simulink model "HARMALYZE_model_simulink"  (R2019b)
settings: Solver=VariableStepAuto  StartTime=0.0  StopTime=2.3  RelTol=1e-3
libraries: powerlib_meascontrol x1
(part 1 of 2)
settings Model: Creator=91850  LastModifiedBy=91850

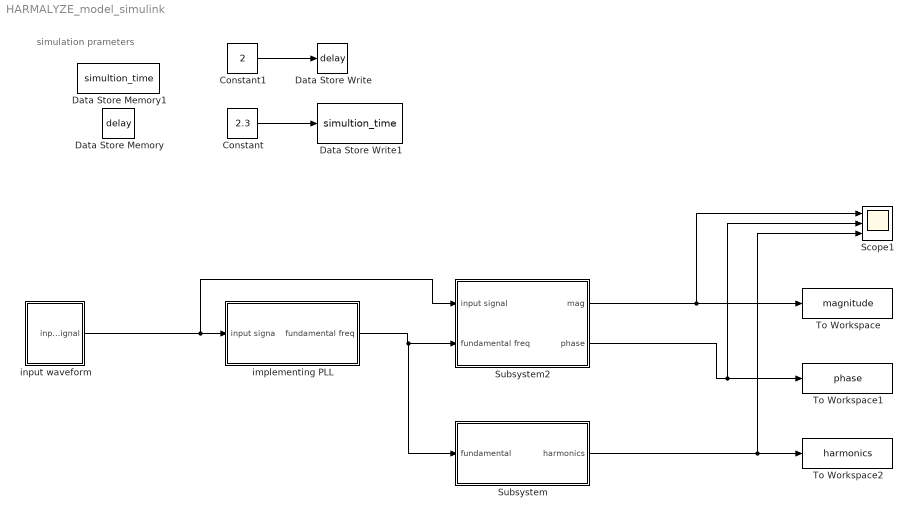
== system HARMALYZE_model_simulink ==
  note: simulation prameters
  Constant : Constant  Value=2.3
  Constant1 : Constant  Value=2
  Data Store Write : DataStoreWrite  DataStoreName=delay
  Data Store Write1 : DataStoreWrite  DataStoreName=simultion_time
  Data Store Memory : DataStoreMemory  DataStoreName=delay  ReadBeforeWriteMsg=warning  WriteAfterWriteMsg=warning  WriteAfterReadMsg=warning  ShowAdditionalParam=off
  Data Store Memory1 : DataStoreMemory  DataStoreName=simultion_time  ReadBeforeWriteMsg=warning  WriteAfterWriteMsg=warning  WriteAfterReadMsg=warning  ShowAdditionalParam=off
  Scope1 : Scope  NumInputPorts=3
  Subsystem : Subsystem
  Subsystem2 : Subsystem
  To Workspace : ToWorkspace  VariableName=magnitude  SaveFormat=Timeseries  SampleTime=-1
  To Workspace1 : ToWorkspace  VariableName=phase  SaveFormat=Timeseries  SampleTime=-1
  To Workspace2 : ToWorkspace  VariableName=harmonics  SaveFormat=Timeseries  SampleTime=-1
  implementing PLL : Subsystem
  input waveform : Subsystem
  wires:
  Constant1/1 -> Data Store Write/1
  Constant/1 -> Data Store Write1/1
  Subsystem2/1("mag ") -> Scope1/1, To Workspace/1
  Subsystem2/2(phase) -> Scope1/2, To Workspace1/1
  input waveform/1(input signal) -> Subsystem2/1(input signal), implementing PLL/1(input signa)
  implementing PLL/1(fundamental freq) -> Subsystem/1(fundamental), Subsystem2/2(fundamental freq)
  Subsystem/1(harmonics) -> Scope1/3, To Workspace2/1

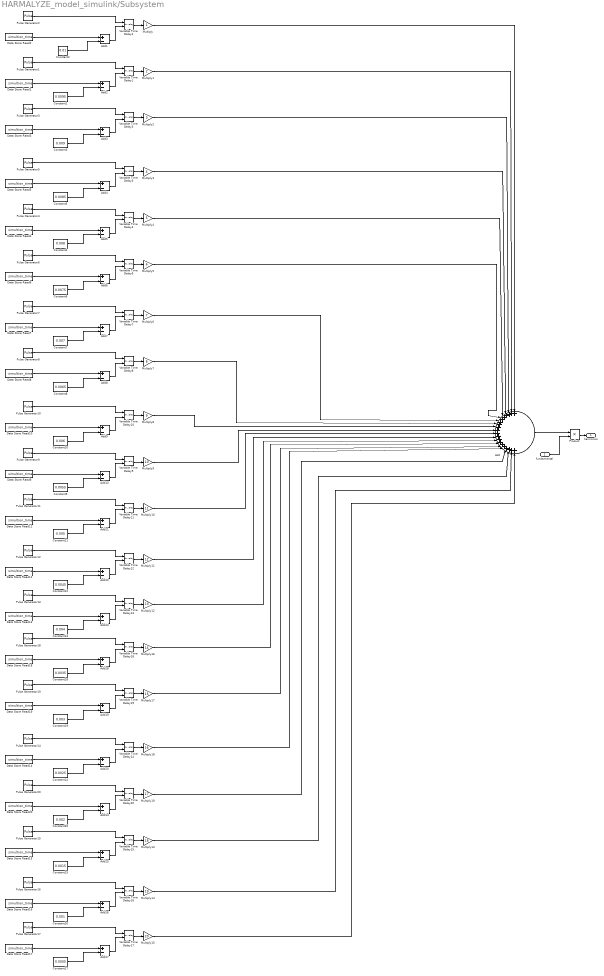
== system HARMALYZE_model_simulink/Subsystem ==
  fundamental : Inport
  Add : Sum  Inputs=20
  Add{1..20} (20 alike) : Sum  Inputs=+-
  Constant1 : Constant  Value=0.0095
  Constant10 : Constant  Value=0.006
  Constant11 : Constant  Value=0.005
  Constant12 : Constant  Value=0.0045
  Constant13 : Constant  Value=0.004
  Constant14 : Constant  Value=0.0025
  Constant15 : Constant  Value=0.0015
  Constant16 : Constant  Value=0.001
  Constant17 : Constant  Value=0.0005
  Constant18 : Constant  Value=0.0035
  Constant19 : Constant  Value=0.003
  Constant2 : Constant  Value=0.01
  Constant20 : Constant  Value=0.002
  Constant3 : Constant  Value=0.009
  Constant4 : Constant  Value=0.008
  Constant5 : Constant  Value=0.0085
  Constant6 : Constant  Value=0.0075
  Constant7 : Constant  Value=0.007
  Constant8 : Constant  Value=0.0065
  Constant9 : Constant  Value=0.0055
  Data Store Read{1..20} (20 alike) : DataStoreRead  DataStoreName=simultion_time
  Multiply : Gain
  Multiply1 : Gain  Gain=2
  Multiply10 : Gain  Gain=11
  Multiply11 : Gain  Gain=12
  Multiply12 : Gain  Gain=13
  Multiply13 : Gain  Gain=18
  Multiply14 : Gain  Gain=19
  Multiply15 : Gain  Gain=20
  Multiply16 : Gain  Gain=14
  Multiply17 : Gain  Gain=15
  Multiply18 : Gain  Gain=16
  Multiply19 : Gain  Gain=17
  Multiply2 : Gain  Gain=3
  Multiply3 : Gain  Gain=4
  Multiply4 : Gain  Gain=5
  Multiply5 : Gain  Gain=6
  Multiply6 : Gain  Gain=7
  Multiply7 : Gain  Gain=8
  Multiply8 : Gain  Gain=9
  Multiply9 : Gain  Gain=10
  Product : Product
  Pulse Generator{1..20} (20 alike) : DiscretePulseGenerator  PulseType=Time based  Period=1  PulseWidth=0.01
  Variable Time Delay{1..20} (20 alike) : VariableTransportDelay  MaximumDelay=10
  harmonics : Outport
  wires:
  Add1/1 -> Variable Time Delay2/2
  Data Store Read2/1 -> Add1/1
  Pulse Generator2/1 -> Variable Time Delay2/1
  Product/1 -> harmonics/1
  Constant2/1 -> Add1/2
  Constant1/1 -> Add2/2
  Pulse Generator1/1 -> Variable Time Delay1/1
  Data Store Read1/1 -> Add2/1
  Add2/1 -> Variable Time Delay1/2
  Add/1 -> Product/1
  fundamental/1 -> Product/2
  Variable Time Delay2/1 -> Multiply/1
  Variable Time Delay1/1 -> Multiply1/1
  Variable Time Delay3/1 -> Multiply2/1
  Add3/1 -> Variable Time Delay3/2
  Data Store Read3/1 -> Add3/1
  Pulse Generator3/1 -> Variable Time Delay3/1
  Constant3/1 -> Add3/2
  Constant6/1 -> Add6/2
  Pulse Generator6/1 -> Variable Time Delay6/1
  Data Store Read6/1 -> Add6/1
  Add6/1 -> Variable Time Delay6/2
  Variable Time Delay6/1 -> Multiply5/1
  Variable Time Delay4/1 -> Multiply4/1
  Variable Time Delay5/1 -> Multiply3/1
  Add5/1 -> Variable Time Delay4/2
  Data Store Read4/1 -> Add5/1
  Pulse Generator4/1 -> Variable Time Delay4/1
  Constant4/1 -> Add5/2
  Constant5/1 -> Add4/2
  Pulse Generator5/1 -> Variable Time Delay5/1
  Data Store Read5/1 -> Add4/1
  Add4/1 -> Variable Time Delay5/2
  Add9/1 -> Variable Time Delay10/2
  Data Store Read10/1 -> Add9/1
  Pulse Generator10/1 -> Variable Time Delay10/1
  Constant10/1 -> Add9/2
  Constant9/1 -> Add10/2
  Pulse Generator9/1 -> Variable Time Delay9/1
  Data Store Read9/1 -> Add10/1
  Add10/1 -> Variable Time Delay9/2
  Variable Time Delay10/1 -> Multiply8/1
  Variable Time Delay9/1 -> Multiply9/1
  Variable Time Delay11/1 -> Multiply10/1
  Add11/1 -> Variable Time Delay11/2
  Data Store Read11/1 -> Add11/1
  Pulse Generator11/1 -> Variable Time Delay11/1
  Constant11/1 -> Add11/2
  Constant8/1 -> Add8/2
  Pulse Generator8/1 -> Variable Time Delay8/1
  Data Store Read8/1 -> Add8/1
  Add8/1 -> Variable Time Delay8/2
  Variable Time Delay8/1 -> Multiply7/1
  Variable Time Delay7/1 -> Multiply6/1
  Add7/1 -> Variable Time Delay7/2
  Data Store Read7/1 -> Add7/1
  Pulse Generator7/1 -> Variable Time Delay7/1
  Constant7/1 -> Add7/2
  Constant12/1 -> Add12/2
  Pulse Generator12/1 -> Variable Time Delay12/1
  Data Store Read12/1 -> Add12/1
  Add12/1 -> Variable Time Delay12/2
  Variable Time Delay12/1 -> Multiply11/1
  Variable Time Delay13/1 -> Multiply12/1
  Add13/1 -> Variable Time Delay13/2
  Data Store Read13/1 -> Add13/1
  Pulse Generator13/1 -> Variable Time Delay13/1
  Constant13/1 -> Add13/2
  Constant17/1 -> Add17/2
  Pulse Generator17/1 -> Variable Time Delay17/1
  Data Store Read17/1 -> Add17/1
  Add17/1 -> Variable Time Delay17/2
  Variable Time Delay17/1 -> Multiply15/1
  Variable Time Delay16/1 -> Multiply14/1
  Add16/1 -> Variable Time Delay16/2
  Data Store Read16/1 -> Add16/1
  Pulse Generator16/1 -> Variable Time Delay16/1
  Constant16/1 -> Add16/2
  Constant18/1 -> Add18/2
  Pulse Generator18/1 -> Variable Time Delay18/1
  Data Store Read18/1 -> Add18/1
  Add18/1 -> Variable Time Delay18/2
  Variable Time Delay18/1 -> Multiply16/1
  Variable Time Delay19/1 -> Multiply17/1
  Add19/1 -> Variable Time Delay19/2
  Data Store Read19/1 -> Add19/1
  Pulse Generator19/1 -> Variable Time Delay19/1
  Constant19/1 -> Add19/2
  Constant15/1 -> Add15/2
  Pulse Generator15/1 -> Variable Time Delay15/1
  Data Store Read15/1 -> Add15/1
  Add15/1 -> Variable Time Delay15/2
  Variable Time Delay15/1 -> Multiply13/1
  Variable Time Delay20/1 -> Multiply19/1
  Variable Time Delay14/1 -> Multiply18/1
  Add14/1 -> Variable Time Delay20/2
  Data Store Read20/1 -> Add14/1
  Pulse Generator20/1 -> Variable Time Delay20/1
  Constant20/1 -> Add14/2
  Constant14/1 -> Add20/2
  Pulse Generator14/1 -> Variable Time Delay14/1
  Data Store Read14/1 -> Add20/1
  Add20/1 -> Variable Time Delay14/2
  Multiply/1 -> Add/1
  Multiply1/1 -> Add/2
  Multiply2/1 -> Add/3
  Multiply3/1 -> Add/4
  Multiply4/1 -> Add/5
  Multiply5/1 -> Add/6
  Multiply6/1 -> Add/7
  Multiply7/1 -> Add/8
  Multiply8/1 -> Add/9
  Multiply9/1 -> Add/10
  Multiply10/1 -> Add/11
  Multiply11/1 -> Add/12
  Multiply12/1 -> Add/13
  Multiply16/1 -> Add/14
  Multiply17/1 -> Add/15
  Multiply18/1 -> Add/16
  Multiply19/1 -> Add/17
  Multiply13/1 -> Add/18
  Multiply14/1 -> Add/19
  Multiply15/1 -> Add/20

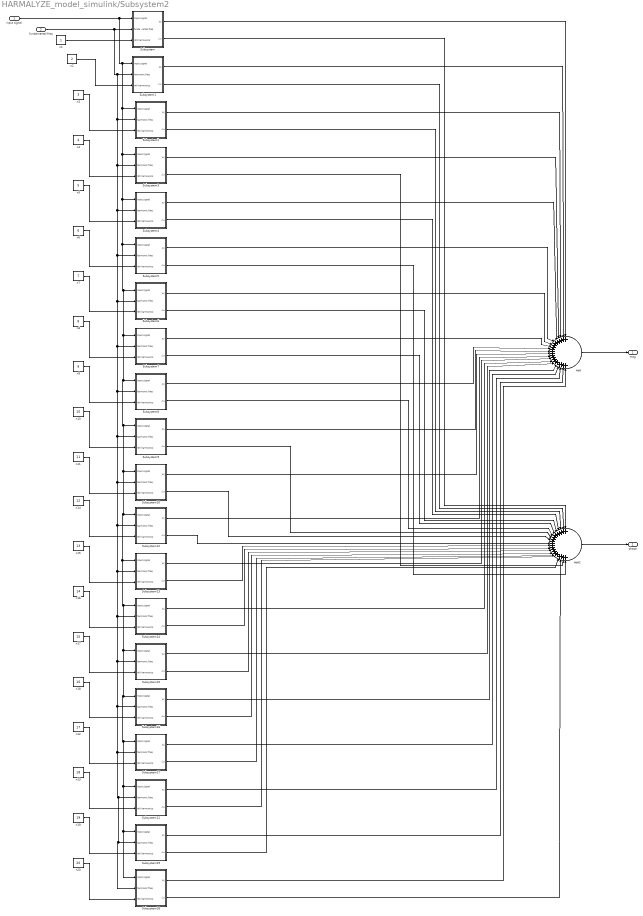
== system HARMALYZE_model_simulink/Subsystem2 ==
  input signal : Inport
  fundamental freq : Inport  Port=2
  Add : Sum  Inputs=20
  Add2 : Sum  Inputs=20
  Subsystem : Subsystem
  Subsystem1 : Subsystem
  Subsystem10 : Subsystem
  Subsystem11 : Subsystem
  Subsystem12 : Subsystem
  Subsystem13 : Subsystem
  Subsystem14 : Subsystem
  Subsystem15 : Subsystem
  Subsystem16 : Subsystem
  Subsystem17 : Subsystem
  Subsystem18 : Subsystem
  Subsystem19 : Subsystem
  Subsystem2 : Subsystem
  Subsystem3 : Subsystem
  Subsystem4 : Subsystem
  Subsystem5 : Subsystem
  Subsystem6 : Subsystem
  Subsystem7 : Subsystem
  Subsystem8 : Subsystem
  Subsystem9 : Subsystem
  n1 : Constant
  n10 : Constant  Value=10
  n11 : Constant  Value=11
  n12 : Constant  Value=17
  n13 : Constant  Value=18
  n14 : Constant  Value=12
  n15 : Constant  Value=13
  n16 : Constant  Value=14
  n17 : Constant  Value=15
  n18 : Constant  Value=16
  n19 : Constant  Value=19
  n2 : Constant  Value=2
  n20 : Constant  Value=20
  n3 : Constant  Value=3
  n4 : Constant  Value=4
  n5 : Constant  Value=5
  n6 : Constant  Value=6
  n7 : Constant  Value=7
  n8 : Constant  Value=8
  n9 : Constant  Value=9
  "mag " : Outport
  phase : Outport  Port=2
  wires:
  Subsystem/1(|u|) -> Add/1
  n1/1 -> Subsystem/3(nth harmonics)
  n2/1 -> Subsystem1/3(nth harmonics)
  Subsystem1/1(|u|) -> Add/2
  Subsystem2/1(|u|) -> Add/3
  n3/1 -> Subsystem2/3(nth harmonics)
  n4/1 -> Subsystem3/3(nth harmonics)
  Subsystem3/1(|u|) -> Add/4
  n5/1 -> Subsystem4/3(nth harmonics)
  Subsystem4/1(|u|) -> Add/5
  n6/1 -> Subsystem5/3(nth harmonics)
  Subsystem5/1(|u|) -> Add/6
  n7/1 -> Subsystem6/3(nth harmonics)
  Subsystem6/1(|u|) -> Add/7
  n8/1 -> Subsystem7/3(nth harmonics)
  Subsystem7/1(|u|) -> Add/8
  n11/1 -> Subsystem10/3(nth harmonics)
  Subsystem9/1(|u|) -> Add/10
  n10/1 -> Subsystem9/3(nth harmonics)
  Subsystem8/1(|u|) -> Add/9
  n9/1 -> Subsystem8/3(nth harmonics)
  n18/1 -> Subsystem16/3(nth harmonics)
  Subsystem16/1(|u|) -> Add/16
  n12/1 -> Subsystem17/3(nth harmonics)
  n13/1 -> Subsystem11/3(nth harmonics)
  Subsystem15/1(|u|) -> Add/15
  n17/1 -> Subsystem15/3(nth harmonics)
  Subsystem14/1(|u|) -> Add/14
  n16/1 -> Subsystem14/3(nth harmonics)
  Subsystem13/1(|u|) -> Add/13
  n15/1 -> Subsystem13/3(nth harmonics)
  Subsystem12/1(|u|) -> Add/12
  n14/1 -> Subsystem12/3(nth harmonics)
  fundamental freq/1 -> Subsystem9/2(harmonic freq), Subsystem13/2(harmonic freq), Subsystem14/2(harmonic freq), Subsystem15/2(harmonic freq), Subsystem16/2(harmonic freq), Subsystem18/2(harmonic freq), Subsystem19/2(harmonic freq), Subsystem11/2(harmonic freq), Subsystem17/2(harmonic freq), Subsystem12/2(harmonic freq), Subsystem10/2(harmonic freq), Subsystem8/2(harmonic freq), Subsystem7/2(harmonic freq), Subsystem6/2(harmonic freq), Subsystem5/2(harmonic freq), Subsystem4/2(harmonic freq), Subsystem3/2(harmonic freq), Subsystem2/2(harmonic freq), Subsystem1/2(harmonic freq), Subsystem/2(fundamental freq)
  n20/1 -> Subsystem18/3(nth harmonics)
  input signal/1 -> Subsystem9/1(input signal), Subsystem13/1(input signal), Subsystem14/1(input signal), Subsystem15/1(input signal), Subsystem16/1(input signal), Subsystem19/1(input signal), Subsystem18/1(input signal), Subsystem11/1(input signal), Subsystem17/1(input signal), Subsystem12/1(input signal), Subsystem10/1(input signal), Subsystem8/1(input signal), Subsystem7/1(input signal), Subsystem6/1(input signal), Subsystem5/1(input signal), Subsystem4/1(input signal), Subsystem3/1(input signal), Subsystem2/1(input signal), Subsystem1/1(input signal), Subsystem/1(input signal)
  n19/1 -> Subsystem19/3(nth harmonics)
  Subsystem10/1(|u|) -> Add/11
  Subsystem17/1(|u|) -> Add/17
  Subsystem11/1(|u|) -> Add/18
  Subsystem19/1(|u|) -> Add/19
  Subsystem18/1(|u|) -> Add/20
  Subsystem/2(∠u) -> Add2/1
  Subsystem1/2(∠u) -> Add2/2
  Subsystem2/2(∠u) -> Add2/3
  Subsystem4/2(∠u) -> Add2/4
  Subsystem6/2(∠u) -> Add2/5
  Subsystem9/2(∠u) -> Add2/8
  Subsystem12/2(∠u) -> Add2/10
  Subsystem10/2(∠u) -> Add2/9
  Subsystem7/2(∠u) -> Add2/6
  Subsystem8/2(∠u) -> Add2/7
  Subsystem13/2(∠u) -> Add2/11
  Subsystem14/2(∠u) -> Add2/12
  Subsystem15/2(∠u) -> Add2/13
  Subsystem16/2(∠u) -> Add2/14
  Subsystem17/2(∠u) -> Add2/15
  Subsystem11/2(∠u) -> Add2/16
  Subsystem19/2(∠u) -> Add2/17
  Subsystem18/2(∠u) -> Add2/18
  Subsystem3/2(∠u) -> Add2/19
  Subsystem5/2(∠u) -> Add2/20
  Add/1 -> "mag "/1
  Add2/1 -> phase/1

== system HARMALYZE_model_simulink/implementing PLL ==
  input signa : Inport
  Clock1 : Clock
  Data Store Read : DataStoreRead  DataStoreName=delay
  If Action Subsystem : Subsystem  TreatAsAtomicUnit=on
  If1 : If  NumInputs=2  IfExpression=u1 == u2  ShowElse=off
  pll : powerlib_meascontrol/PLL/PLL  Fmin=10  Par_Init=[0, 40]  ParK=[180, 3200, 1]  TcD=1e-4  MaxRateChangeFreq=10  FilterCutOffFreq=25  Ts=0  AGC=on
      settings: SourceProductName=Simscape Electrical  SourceProductBaseCode=PS
  fundamental freq : Outport
  wires:
  If Action Subsystem/1(Out1) -> fundamental freq/1
  If1/1 -> If Action Subsystem/Action
  Clock1/1 -> If1/1
  pll/1 -> If Action Subsystem/1(In1)
  Data Store Read/1 -> If1/2
  input signa/1 -> pll/1

== system HARMALYZE_model_simulink/input waveform ==
  Add1 : Sum  Inputs=5
  "fundamental " : SignalGenerator  Amplitude=10  Frequency=50
  harmonic 1 : SignalGenerator  Amplitude=5  Frequency=100
  harmonic 2 : SignalGenerator  Amplitude=3  Frequency=150
  harmonic 3 : SignalGenerator  Amplitude=2  Frequency=200
  harmonic 4 : SignalGenerator  Frequency=250
  input signal : Outport
  wires:
  harmonic 1/1 -> Add1/2
  harmonic 2/1 -> Add1/3
  Add1/1 -> input signal/1
  "fundamental "/1 -> Add1/1
  harmonic 3/1 -> Add1/4
  harmonic 4/1 -> Add1/5

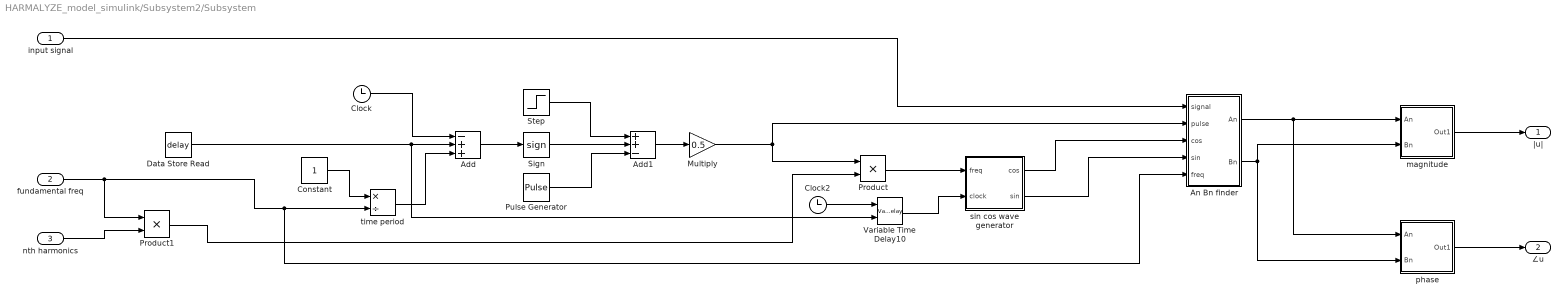
== system HARMALYZE_model_simulink/Subsystem2/Subsystem ==
  input signal : Inport
  fundamental freq : Inport  Port=2
  nth harmonics : Inport  Port=3
  Add : Sum  Inputs=-++
  Add1 : Sum  Inputs=++-
  An Bn finder : Subsystem
  Clock : Clock
  Clock2 : Clock
  Constant : Constant
  Data Store Read : DataStoreRead  DataStoreName=delay
  Multiply : Gain  Gain=0.5
  Product : Product
  Product1 : Product
  Pulse Generator : DiscretePulseGenerator  PulseType=Time based  Period=4  PulseWidth=50
  Sign : Signum
  Step : Step  Time=2  SampleTime=0
  Variable Time Delay10 : VariableTransportDelay  MaximumDelay=10
  magnitude : Subsystem
  phase : Subsystem
  sin cos wave generator : Subsystem
  "time period " : Product  Inputs=*/
  |u| : Outport
  ∠u : Outport  Port=2
  wires:
  input signal/1 -> An Bn finder/1(signal)
  sin cos wave generator/2(sin) -> An Bn finder/4(sin)
  sin cos wave generator/1(cos) -> An Bn finder/3(cos)
  Variable Time Delay10/1 -> sin cos wave generator/2(clock)
  "time period "/1 -> Add/3
  Data Store Read/1 -> Variable Time Delay10/2, Add/2
  Multiply/1 -> Product/1, An Bn finder/2(pulse)
  Product/1 -> sin cos wave generator/1(freq)
  Clock/1 -> Add/1
  Add/1 -> Sign/1
  Constant/1 -> "time period "/1
  Step/1 -> Add1/1
  Sign/1 -> Add1/2
  Pulse Generator/1 -> Add1/3
  Clock2/1 -> Variable Time Delay10/1
  Add1/1 -> Multiply/1
  Product1/1 -> Product/2
  An Bn finder/2(Bn) -> phase/2(Bn), magnitude/2(Bn)
  An Bn finder/1(An) -> phase/1(An), magnitude/1(An)
  magnitude/1(Out1) -> |u|/1
  phase/1(Out1) -> ∠u/1
  nth harmonics/1 -> Product1/2
  fundamental freq/1 -> Product1/1, An Bn finder/5("freq "), "time period "/2

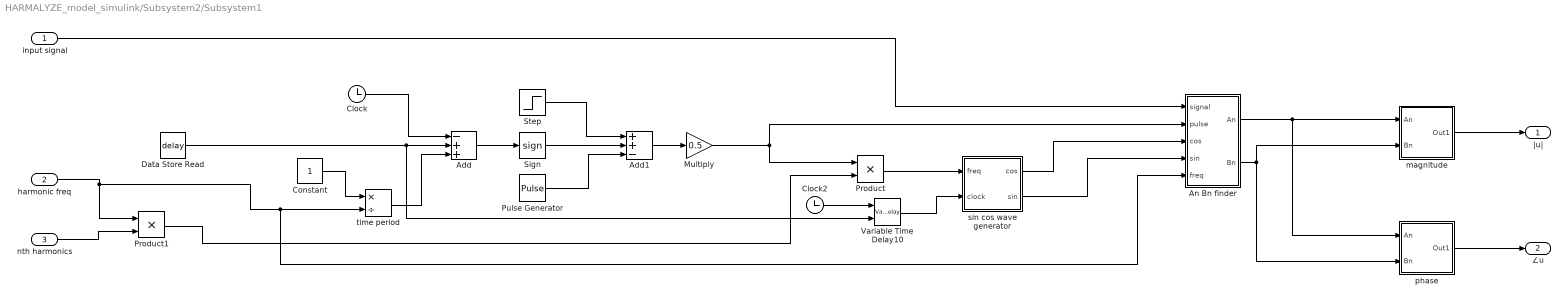
== system HARMALYZE_model_simulink/Subsystem2/Subsystem1 ==
  input signal : Inport
  harmonic freq : Inport  Port=2
  nth harmonics : Inport  Port=3
  Add : Sum  Inputs=-++
  Add1 : Sum  Inputs=++-
  An Bn finder : Subsystem
  Clock : Clock
  Clock2 : Clock
  Constant : Constant
  Data Store Read : DataStoreRead  DataStoreName=delay
  Multiply : Gain  Gain=0.5
  Product : Product
  Product1 : Product
  Pulse Generator : DiscretePulseGenerator  PulseType=Time based  Period=4  PulseWidth=50
  Sign : Signum
  Step : Step  Time=2  SampleTime=0
  Variable Time Delay10 : VariableTransportDelay  MaximumDelay=10
  magnitude : Subsystem
  phase : Subsystem
  sin cos wave generator : Subsystem
  "time period " : Product  Inputs=*/
  |u| : Outport
  ∠u : Outport  Port=2
  wires:
  harmonic freq/1 -> Product1/1, "time period "/2, An Bn finder/5("freq ")
  nth harmonics/1 -> Product1/2
  phase/1(Out1) -> ∠u/1
  magnitude/1(Out1) -> |u|/1
  An Bn finder/1(An) -> magnitude/1(An), phase/1(An)
  An Bn finder/2(Bn) -> magnitude/2(Bn), phase/2(Bn)
  Product1/1 -> Product/2
  Add1/1 -> Multiply/1
  Clock2/1 -> Variable Time Delay10/1
  Pulse Generator/1 -> Add1/3
  Sign/1 -> Add1/2
  Step/1 -> Add1/1
  Constant/1 -> "time period "/1
  Add/1 -> Sign/1
  Clock/1 -> Add/1
  Product/1 -> sin cos wave generator/1(freq)
  Multiply/1 -> An Bn finder/2(pulse), Product/1
  Data Store Read/1 -> Add/2, Variable Time Delay10/2
  "time period "/1 -> Add/3
  Variable Time Delay10/1 -> sin cos wave generator/2(clock)
  sin cos wave generator/1(cos) -> An Bn finder/3(cos)
  sin cos wave generator/2(sin) -> An Bn finder/4(sin)
  input signal/1 -> An Bn finder/1(signal)

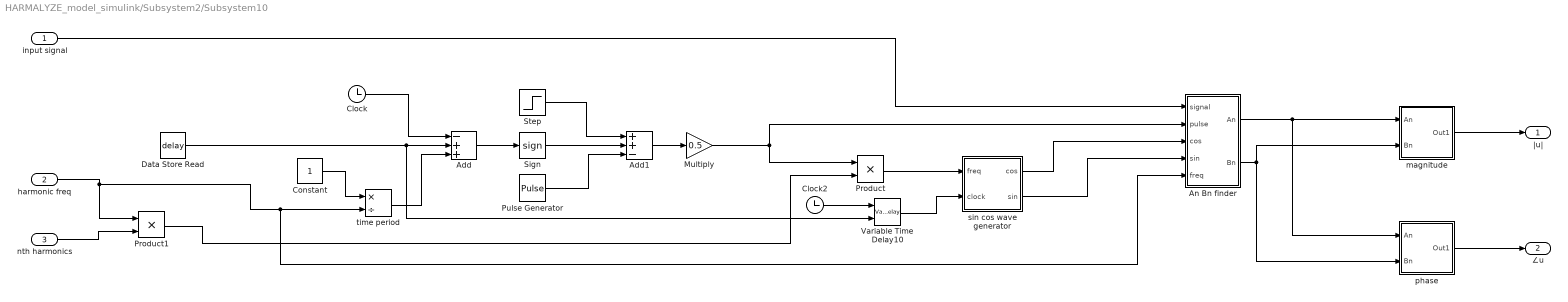
== system HARMALYZE_model_simulink/Subsystem2/Subsystem10 ==
  input signal : Inport
  harmonic freq : Inport  Port=2
  nth harmonics : Inport  Port=3
  Add : Sum  Inputs=-++
  Add1 : Sum  Inputs=++-
  An Bn finder : Subsystem
  Clock : Clock
  Clock2 : Clock
  Constant : Constant
  Data Store Read : DataStoreRead  DataStoreName=delay
  Multiply : Gain  Gain=0.5
  Product : Product
  Product1 : Product
  Pulse Generator : DiscretePulseGenerator  PulseType=Time based  Period=4  PulseWidth=50
  Sign : Signum
  Step : Step  Time=2  SampleTime=0
  Variable Time Delay10 : VariableTransportDelay  MaximumDelay=10
  magnitude : Subsystem
  phase : Subsystem
  sin cos wave generator : Subsystem
  "time period " : Product  Inputs=*/
  |u| : Outport
  ∠u : Outport  Port=2
  wires:
  harmonic freq/1 -> Product1/1, "time period "/2, An Bn finder/5("freq ")
  nth harmonics/1 -> Product1/2
  phase/1(Out1) -> ∠u/1
  magnitude/1(Out1) -> |u|/1
  An Bn finder/1(An) -> magnitude/1(An), phase/1(An)
  An Bn finder/2(Bn) -> magnitude/2(Bn), phase/2(Bn)
  Product1/1 -> Product/2
  Add1/1 -> Multiply/1
  Clock2/1 -> Variable Time Delay10/1
  Pulse Generator/1 -> Add1/3
  Sign/1 -> Add1/2
  Step/1 -> Add1/1
  Constant/1 -> "time period "/1
  Add/1 -> Sign/1
  Clock/1 -> Add/1
  Product/1 -> sin cos wave generator/1(freq)
  Multiply/1 -> An Bn finder/2(pulse), Product/1
  Data Store Read/1 -> Add/2, Variable Time Delay10/2
  "time period "/1 -> Add/3
  Variable Time Delay10/1 -> sin cos wave generator/2(clock)
  sin cos wave generator/1(cos) -> An Bn finder/3(cos)
  sin cos wave generator/2(sin) -> An Bn finder/4(sin)
  input signal/1 -> An Bn finder/1(signal)

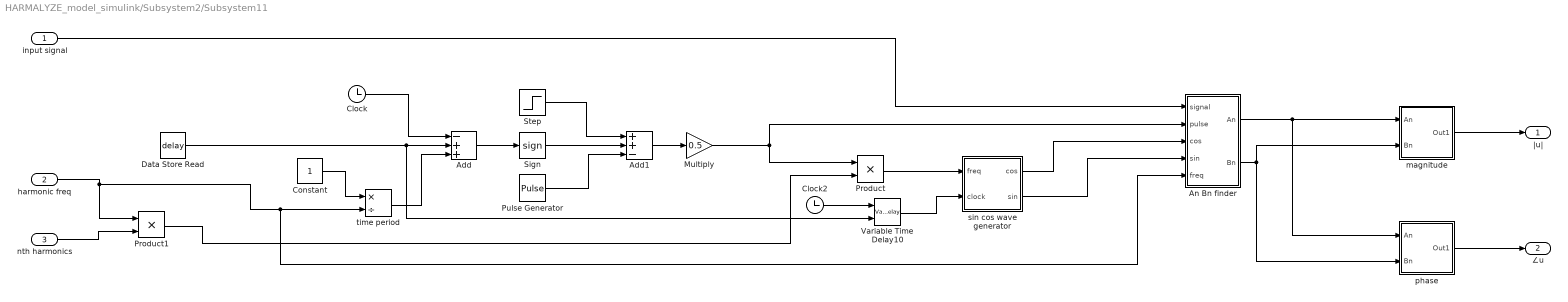
== system HARMALYZE_model_simulink/Subsystem2/Subsystem11 ==
  input signal : Inport
  harmonic freq : Inport  Port=2
  nth harmonics : Inport  Port=3
  Add : Sum  Inputs=-++
  Add1 : Sum  Inputs=++-
  An Bn finder : Subsystem
  Clock : Clock
  Clock2 : Clock
  Constant : Constant
  Data Store Read : DataStoreRead  DataStoreName=delay
  Multiply : Gain  Gain=0.5
  Product : Product
  Product1 : Product
  Pulse Generator : DiscretePulseGenerator  PulseType=Time based  Period=4  PulseWidth=50
  Sign : Signum
  Step : Step  Time=2  SampleTime=0
  Variable Time Delay10 : VariableTransportDelay  MaximumDelay=10
  magnitude : Subsystem
  phase : Subsystem
  sin cos wave generator : Subsystem
  "time period " : Product  Inputs=*/
  |u| : Outport
  ∠u : Outport  Port=2
  wires:
  input signal/1 -> An Bn finder/1(signal)
  sin cos wave generator/2(sin) -> An Bn finder/4(sin)
  sin cos wave generator/1(cos) -> An Bn finder/3(cos)
  Variable Time Delay10/1 -> sin cos wave generator/2(clock)
  "time period "/1 -> Add/3
  Data Store Read/1 -> Variable Time Delay10/2, Add/2
  Multiply/1 -> Product/1, An Bn finder/2(pulse)
  Product/1 -> sin cos wave generator/1(freq)
  Clock/1 -> Add/1
  Add/1 -> Sign/1
  Constant/1 -> "time period "/1
  Step/1 -> Add1/1
  Sign/1 -> Add1/2
  Pulse Generator/1 -> Add1/3
  Clock2/1 -> Variable Time Delay10/1
  Add1/1 -> Multiply/1
  Product1/1 -> Product/2
  An Bn finder/2(Bn) -> phase/2(Bn), magnitude/2(Bn)
  An Bn finder/1(An) -> phase/1(An), magnitude/1(An)
  magnitude/1(Out1) -> |u|/1
  phase/1(Out1) -> ∠u/1
  nth harmonics/1 -> Product1/2
  harmonic freq/1 -> An Bn finder/5("freq "), "time period "/2, Product1/1

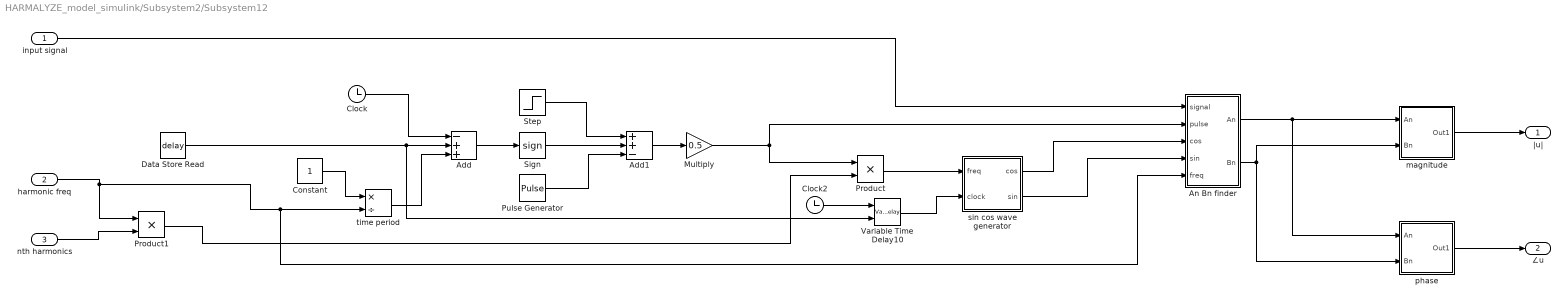
== system HARMALYZE_model_simulink/Subsystem2/Subsystem12 ==
  input signal : Inport
  harmonic freq : Inport  Port=2
  nth harmonics : Inport  Port=3
  Add : Sum  Inputs=-++
  Add1 : Sum  Inputs=++-
  An Bn finder : Subsystem
  Clock : Clock
  Clock2 : Clock
  Constant : Constant
  Data Store Read : DataStoreRead  DataStoreName=delay
  Multiply : Gain  Gain=0.5
  Product : Product
  Product1 : Product
  Pulse Generator : DiscretePulseGenerator  PulseType=Time based  Period=4  PulseWidth=50
  Sign : Signum
  Step : Step  Time=2  SampleTime=0
  Variable Time Delay10 : VariableTransportDelay  MaximumDelay=10
  magnitude : Subsystem
  phase : Subsystem
  sin cos wave generator : Subsystem
  "time period " : Product  Inputs=*/
  |u| : Outport
  ∠u : Outport  Port=2
  wires:
  harmonic freq/1 -> Product1/1, "time period "/2, An Bn finder/5("freq ")
  nth harmonics/1 -> Product1/2
  phase/1(Out1) -> ∠u/1
  magnitude/1(Out1) -> |u|/1
  An Bn finder/1(An) -> magnitude/1(An), phase/1(An)
  An Bn finder/2(Bn) -> magnitude/2(Bn), phase/2(Bn)
  Product1/1 -> Product/2
  Add1/1 -> Multiply/1
  Clock2/1 -> Variable Time Delay10/1
  Pulse Generator/1 -> Add1/3
  Sign/1 -> Add1/2
  Step/1 -> Add1/1
  Constant/1 -> "time period "/1
  Add/1 -> Sign/1
  Clock/1 -> Add/1
  Product/1 -> sin cos wave generator/1(freq)
  Multiply/1 -> An Bn finder/2(pulse), Product/1
  Data Store Read/1 -> Add/2, Variable Time Delay10/2
  "time period "/1 -> Add/3
  Variable Time Delay10/1 -> sin cos wave generator/2(clock)
  sin cos wave generator/1(cos) -> An Bn finder/3(cos)
  sin cos wave generator/2(sin) -> An Bn finder/4(sin)
  input signal/1 -> An Bn finder/1(signal)

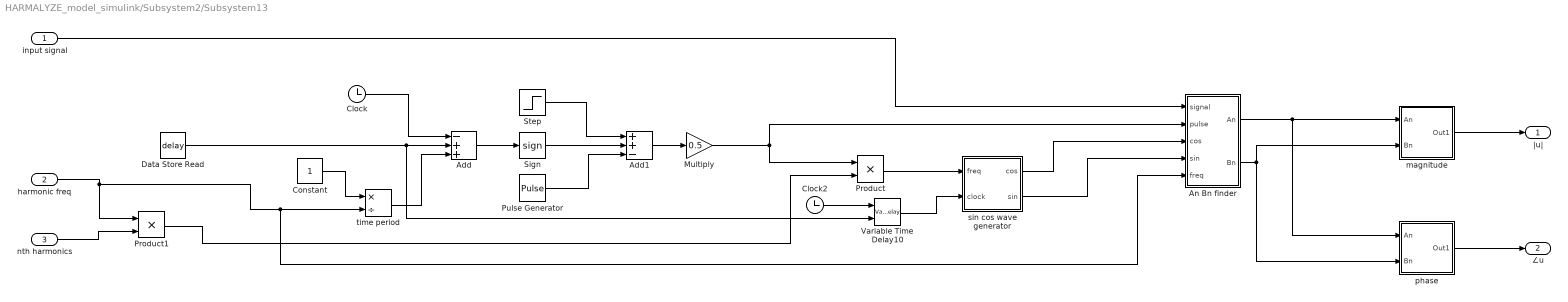
== system HARMALYZE_model_simulink/Subsystem2/Subsystem13 ==
  input signal : Inport
  harmonic freq : Inport  Port=2
  nth harmonics : Inport  Port=3
  Add : Sum  Inputs=-++
  Add1 : Sum  Inputs=++-
  An Bn finder : Subsystem
  Clock : Clock
  Clock2 : Clock
  Constant : Constant
  Data Store Read : DataStoreRead  DataStoreName=delay
  Multiply : Gain  Gain=0.5
  Product : Product
  Product1 : Product
  Pulse Generator : DiscretePulseGenerator  PulseType=Time based  Period=4  PulseWidth=50
  Sign : Signum
  Step : Step  Time=2  SampleTime=0
  Variable Time Delay10 : VariableTransportDelay  MaximumDelay=10
  magnitude : Subsystem
  phase : Subsystem
  sin cos wave generator : Subsystem
  "time period " : Product  Inputs=*/
  |u| : Outport
  ∠u : Outport  Port=2
  wires:
  harmonic freq/1 -> Product1/1, "time period "/2, An Bn finder/5("freq ")
  nth harmonics/1 -> Product1/2
  phase/1(Out1) -> ∠u/1
  magnitude/1(Out1) -> |u|/1
  An Bn finder/1(An) -> magnitude/1(An), phase/1(An)
  An Bn finder/2(Bn) -> magnitude/2(Bn), phase/2(Bn)
  Product1/1 -> Product/2
  Add1/1 -> Multiply/1
  Clock2/1 -> Variable Time Delay10/1
  Pulse Generator/1 -> Add1/3
  Sign/1 -> Add1/2
  Step/1 -> Add1/1
  Constant/1 -> "time period "/1
  Add/1 -> Sign/1
  Clock/1 -> Add/1
  Product/1 -> sin cos wave generator/1(freq)
  Multiply/1 -> An Bn finder/2(pulse), Product/1
  Data Store Read/1 -> Add/2, Variable Time Delay10/2
  "time period "/1 -> Add/3
  Variable Time Delay10/1 -> sin cos wave generator/2(clock)
  sin cos wave generator/1(cos) -> An Bn finder/3(cos)
  sin cos wave generator/2(sin) -> An Bn finder/4(sin)
  input signal/1 -> An Bn finder/1(signal)

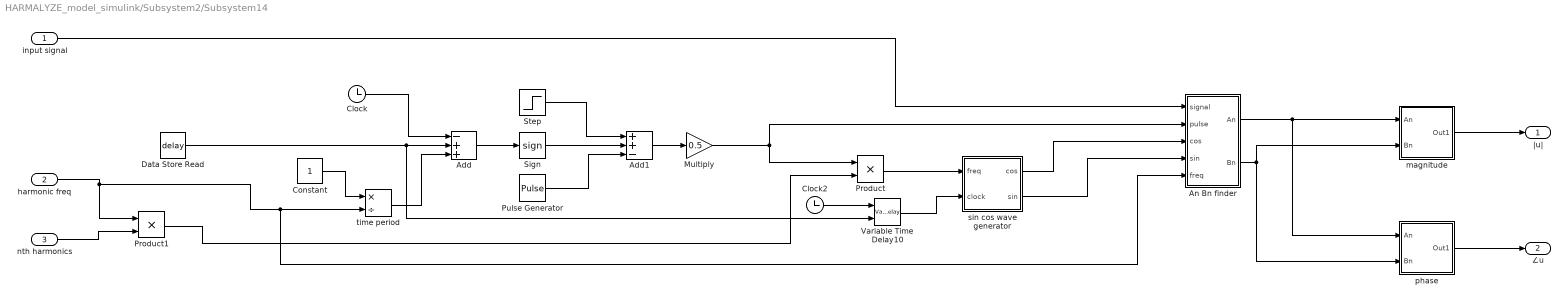
== system HARMALYZE_model_simulink/Subsystem2/Subsystem14 ==
  input signal : Inport
  harmonic freq : Inport  Port=2
  nth harmonics : Inport  Port=3
  Add : Sum  Inputs=-++
  Add1 : Sum  Inputs=++-
  An Bn finder : Subsystem
  Clock : Clock
  Clock2 : Clock
  Constant : Constant
  Data Store Read : DataStoreRead  DataStoreName=delay
  Multiply : Gain  Gain=0.5
  Product : Product
  Product1 : Product
  Pulse Generator : DiscretePulseGenerator  PulseType=Time based  Period=4  PulseWidth=50
  Sign : Signum
  Step : Step  Time=2  SampleTime=0
  Variable Time Delay10 : VariableTransportDelay  MaximumDelay=10
  magnitude : Subsystem
  phase : Subsystem
  sin cos wave generator : Subsystem
  "time period " : Product  Inputs=*/
  |u| : Outport
  ∠u : Outport  Port=2
  wires:
  harmonic freq/1 -> Product1/1, "time period "/2, An Bn finder/5("freq ")
  nth harmonics/1 -> Product1/2
  phase/1(Out1) -> ∠u/1
  magnitude/1(Out1) -> |u|/1
  An Bn finder/1(An) -> magnitude/1(An), phase/1(An)
  An Bn finder/2(Bn) -> magnitude/2(Bn), phase/2(Bn)
  Product1/1 -> Product/2
  Add1/1 -> Multiply/1
  Clock2/1 -> Variable Time Delay10/1
  Pulse Generator/1 -> Add1/3
  Sign/1 -> Add1/2
  Step/1 -> Add1/1
  Constant/1 -> "time period "/1
  Add/1 -> Sign/1
  Clock/1 -> Add/1
  Product/1 -> sin cos wave generator/1(freq)
  Multiply/1 -> An Bn finder/2(pulse), Product/1
  Data Store Read/1 -> Add/2, Variable Time Delay10/2
  "time period "/1 -> Add/3
  Variable Time Delay10/1 -> sin cos wave generator/2(clock)
  sin cos wave generator/1(cos) -> An Bn finder/3(cos)
  sin cos wave generator/2(sin) -> An Bn finder/4(sin)
  input signal/1 -> An Bn finder/1(signal)

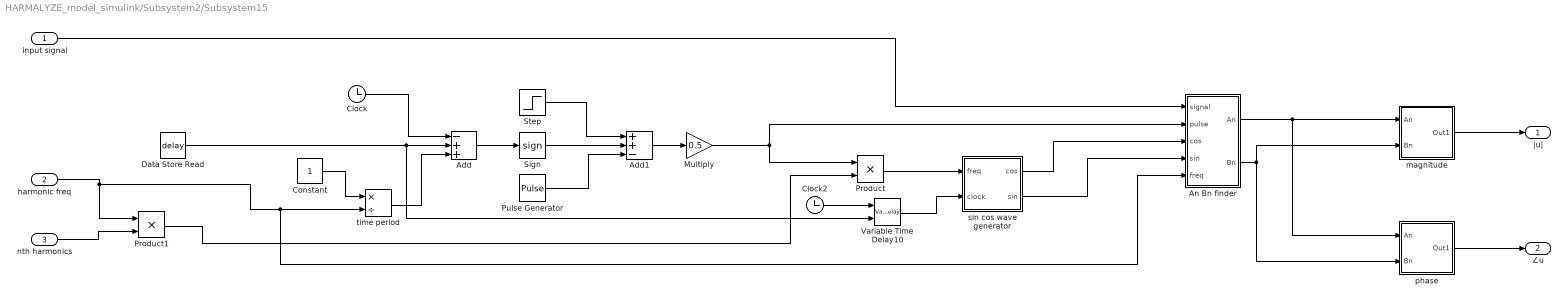
== system HARMALYZE_model_simulink/Subsystem2/Subsystem15 ==
  input signal : Inport
  harmonic freq : Inport  Port=2
  nth harmonics : Inport  Port=3
  Add : Sum  Inputs=-++
  Add1 : Sum  Inputs=++-
  An Bn finder : Subsystem
  Clock : Clock
  Clock2 : Clock
  Constant : Constant
  Data Store Read : DataStoreRead  DataStoreName=delay
  Multiply : Gain  Gain=0.5
  Product : Product
  Product1 : Product
  Pulse Generator : DiscretePulseGenerator  PulseType=Time based  Period=4  PulseWidth=50
  Sign : Signum
  Step : Step  Time=2  SampleTime=0
  Variable Time Delay10 : VariableTransportDelay  MaximumDelay=10
  magnitude : Subsystem
  phase : Subsystem
  sin cos wave generator : Subsystem
  "time period " : Product  Inputs=*/
  |u| : Outport
  ∠u : Outport  Port=2
  wires:
  harmonic freq/1 -> Product1/1, "time period "/2, An Bn finder/5("freq ")
  nth harmonics/1 -> Product1/2
  phase/1(Out1) -> ∠u/1
  magnitude/1(Out1) -> |u|/1
  An Bn finder/1(An) -> magnitude/1(An), phase/1(An)
  An Bn finder/2(Bn) -> magnitude/2(Bn), phase/2(Bn)
  Product1/1 -> Product/2
  Add1/1 -> Multiply/1
  Clock2/1 -> Variable Time Delay10/1
  Pulse Generator/1 -> Add1/3
  Sign/1 -> Add1/2
  Step/1 -> Add1/1
  Constant/1 -> "time period "/1
  Add/1 -> Sign/1
  Clock/1 -> Add/1
  Product/1 -> sin cos wave generator/1(freq)
  Multiply/1 -> An Bn finder/2(pulse), Product/1
  Data Store Read/1 -> Add/2, Variable Time Delay10/2
  "time period "/1 -> Add/3
  Variable Time Delay10/1 -> sin cos wave generator/2(clock)
  sin cos wave generator/1(cos) -> An Bn finder/3(cos)
  sin cos wave generator/2(sin) -> An Bn finder/4(sin)
  input signal/1 -> An Bn finder/1(signal)

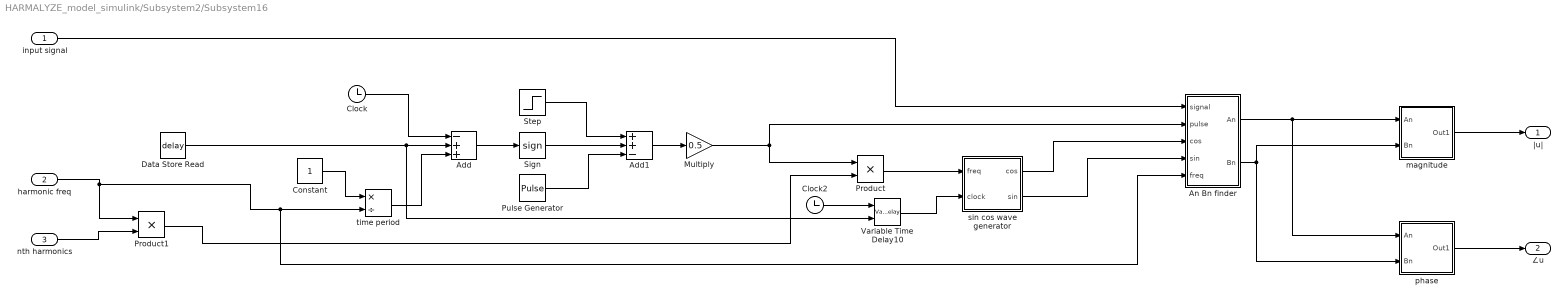
== system HARMALYZE_model_simulink/Subsystem2/Subsystem16 ==
  input signal : Inport
  harmonic freq : Inport  Port=2
  nth harmonics : Inport  Port=3
  Add : Sum  Inputs=-++
  Add1 : Sum  Inputs=++-
  An Bn finder : Subsystem
  Clock : Clock
  Clock2 : Clock
  Constant : Constant
  Data Store Read : DataStoreRead  DataStoreName=delay
  Multiply : Gain  Gain=0.5
  Product : Product
  Product1 : Product
  Pulse Generator : DiscretePulseGenerator  PulseType=Time based  Period=4  PulseWidth=50
  Sign : Signum
  Step : Step  Time=2  SampleTime=0
  Variable Time Delay10 : VariableTransportDelay  MaximumDelay=10
  magnitude : Subsystem
  phase : Subsystem
  sin cos wave generator : Subsystem
  "time period " : Product  Inputs=*/
  |u| : Outport
  ∠u : Outport  Port=2
  wires:
  input signal/1 -> An Bn finder/1(signal)
  sin cos wave generator/2(sin) -> An Bn finder/4(sin)
  sin cos wave generator/1(cos) -> An Bn finder/3(cos)
  Variable Time Delay10/1 -> sin cos wave generator/2(clock)
  "time period "/1 -> Add/3
  Data Store Read/1 -> Variable Time Delay10/2, Add/2
  Multiply/1 -> Product/1, An Bn finder/2(pulse)
  Product/1 -> sin cos wave generator/1(freq)
  Clock/1 -> Add/1
  Add/1 -> Sign/1
  Constant/1 -> "time period "/1
  Step/1 -> Add1/1
  Sign/1 -> Add1/2
  Pulse Generator/1 -> Add1/3
  Clock2/1 -> Variable Time Delay10/1
  Add1/1 -> Multiply/1
  Product1/1 -> Product/2
  An Bn finder/2(Bn) -> phase/2(Bn), magnitude/2(Bn)
  An Bn finder/1(An) -> phase/1(An), magnitude/1(An)
  magnitude/1(Out1) -> |u|/1
  phase/1(Out1) -> ∠u/1
  nth harmonics/1 -> Product1/2
  harmonic freq/1 -> An Bn finder/5("freq "), "time period "/2, Product1/1

== system HARMALYZE_model_simulink/Subsystem2/Subsystem17 ==
  input signal : Inport
  harmonic freq : Inport  Port=2
  nth harmonics : Inport  Port=3
  Add : Sum  Inputs=-++
  Add1 : Sum  Inputs=++-
  An Bn finder : Subsystem
  Clock : Clock
  Clock2 : Clock
  Constant : Constant
  Data Store Read : DataStoreRead  DataStoreName=delay
  Multiply : Gain  Gain=0.5
  Product : Product
  Product1 : Product
  Pulse Generator : DiscretePulseGenerator  PulseType=Time based  Period=4  PulseWidth=50
  Sign : Signum
  Step : Step  Time=2  SampleTime=0
  Variable Time Delay10 : VariableTransportDelay  MaximumDelay=10
  magnitude : Subsystem
  phase : Subsystem
  sin cos wave generator : Subsystem
  "time period " : Product  Inputs=*/
  |u| : Outport
  ∠u : Outport  Port=2
  wires:
  input signal/1 -> An Bn finder/1(signal)
  sin cos wave generator/2(sin) -> An Bn finder/4(sin)
  sin cos wave generator/1(cos) -> An Bn finder/3(cos)
  Variable Time Delay10/1 -> sin cos wave generator/2(clock)
  "time period "/1 -> Add/3
  Data Store Read/1 -> Variable Time Delay10/2, Add/2
  Multiply/1 -> Product/1, An Bn finder/2(pulse)
  Product/1 -> sin cos wave generator/1(freq)
  Clock/1 -> Add/1
  Add/1 -> Sign/1
  Constant/1 -> "time period "/1
  Step/1 -> Add1/1
  Sign/1 -> Add1/2
  Pulse Generator/1 -> Add1/3
  Clock2/1 -> Variable Time Delay10/1
  Add1/1 -> Multiply/1
  Product1/1 -> Product/2
  An Bn finder/2(Bn) -> phase/2(Bn), magnitude/2(Bn)
  An Bn finder/1(An) -> phase/1(An), magnitude/1(An)
  magnitude/1(Out1) -> |u|/1
  phase/1(Out1) -> ∠u/1
  nth harmonics/1 -> Product1/2
  harmonic freq/1 -> An Bn finder/5("freq "), "time period "/2, Product1/1

== system HARMALYZE_model_simulink/Subsystem2/Subsystem18 ==
  input signal : Inport
  harmonic freq : Inport  Port=2
  nth harmonics : Inport  Port=3
  Add : Sum  Inputs=-++
  Add1 : Sum  Inputs=++-
  An Bn finder : Subsystem
  Clock : Clock
  Clock2 : Clock
  Constant : Constant
  Data Store Read : DataStoreRead  DataStoreName=delay
  Multiply : Gain  Gain=0.5
  Product : Product
  Product1 : Product
  Pulse Generator : DiscretePulseGenerator  PulseType=Time based  Period=4  PulseWidth=50
  Sign : Signum
  Step : Step  Time=2  SampleTime=0
  Variable Time Delay10 : VariableTransportDelay  MaximumDelay=10
  magnitude : Subsystem
  phase : Subsystem
  sin cos wave generator : Subsystem
  "time period " : Product  Inputs=*/
  |u| : Outport
  ∠u : Outport  Port=2
  wires:
  harmonic freq/1 -> Product1/1, "time period "/2, An Bn finder/5("freq ")
  nth harmonics/1 -> Product1/2
  phase/1(Out1) -> ∠u/1
  magnitude/1(Out1) -> |u|/1
  An Bn finder/1(An) -> magnitude/1(An), phase/1(An)
  An Bn finder/2(Bn) -> magnitude/2(Bn), phase/2(Bn)
  Product1/1 -> Product/2
  Add1/1 -> Multiply/1
  Clock2/1 -> Variable Time Delay10/1
  Pulse Generator/1 -> Add1/3
  Sign/1 -> Add1/2
  Step/1 -> Add1/1
  Constant/1 -> "time period "/1
  Add/1 -> Sign/1
  Clock/1 -> Add/1
  Product/1 -> sin cos wave generator/1(freq)
  Multiply/1 -> An Bn finder/2(pulse), Product/1
  Data Store Read/1 -> Add/2, Variable Time Delay10/2
  "time period "/1 -> Add/3
  Variable Time Delay10/1 -> sin cos wave generator/2(clock)
  sin cos wave generator/1(cos) -> An Bn finder/3(cos)
  sin cos wave generator/2(sin) -> An Bn finder/4(sin)
  input signal/1 -> An Bn finder/1(signal)

== system HARMALYZE_model_simulink/Subsystem2/Subsystem19 ==
  input signal : Inport
  harmonic freq : Inport  Port=2
  nth harmonics : Inport  Port=3
  Add : Sum  Inputs=-++
  Add1 : Sum  Inputs=++-
  An Bn finder : Subsystem
  Clock : Clock
  Clock2 : Clock
  Constant : Constant
  Data Store Read : DataStoreRead  DataStoreName=delay
  Multiply : Gain  Gain=0.5
  Product : Product
  Product1 : Product
  Pulse Generator : DiscretePulseGenerator  PulseType=Time based  Period=4  PulseWidth=50
  Sign : Signum
  Step : Step  Time=2  SampleTime=0
  Variable Time Delay10 : VariableTransportDelay  MaximumDelay=10
  magnitude : Subsystem
  phase : Subsystem
  sin cos wave generator : Subsystem
  "time period " : Product  Inputs=*/
  |u| : Outport
  ∠u : Outport  Port=2
  wires:
  harmonic freq/1 -> Product1/1, "time period "/2, An Bn finder/5("freq ")
  nth harmonics/1 -> Product1/2
  phase/1(Out1) -> ∠u/1
  magnitude/1(Out1) -> |u|/1
  An Bn finder/1(An) -> magnitude/1(An), phase/1(An)
  An Bn finder/2(Bn) -> magnitude/2(Bn), phase/2(Bn)
  Product1/1 -> Product/2
  Add1/1 -> Multiply/1
  Clock2/1 -> Variable Time Delay10/1
  Pulse Generator/1 -> Add1/3
  Sign/1 -> Add1/2
  Step/1 -> Add1/1
  Constant/1 -> "time period "/1
  Add/1 -> Sign/1
  Clock/1 -> Add/1
  Product/1 -> sin cos wave generator/1(freq)
  Multiply/1 -> An Bn finder/2(pulse), Product/1
  Data Store Read/1 -> Add/2, Variable Time Delay10/2
  "time period "/1 -> Add/3
  Variable Time Delay10/1 -> sin cos wave generator/2(clock)
  sin cos wave generator/1(cos) -> An Bn finder/3(cos)
  sin cos wave generator/2(sin) -> An Bn finder/4(sin)
  input signal/1 -> An Bn finder/1(signal)

== system HARMALYZE_model_simulink/Subsystem2/Subsystem2 ==
  input signal : Inport
  harmonic freq : Inport  Port=2
  nth harmonics : Inport  Port=3
  Add : Sum  Inputs=-++
  Add1 : Sum  Inputs=++-
  An Bn finder : Subsystem
  Clock : Clock
  Clock2 : Clock
  Constant : Constant
  Data Store Read : DataStoreRead  DataStoreName=delay
  Multiply : Gain  Gain=0.5
  Product : Product
  Product1 : Product
  Pulse Generator : DiscretePulseGenerator  PulseType=Time based  Period=4  PulseWidth=50
  Sign : Signum
  Step : Step  Time=2  SampleTime=0
  Variable Time Delay10 : VariableTransportDelay  MaximumDelay=10
  magnitude : Subsystem
  phase : Subsystem
  sin cos wave generator : Subsystem
  "time period " : Product  Inputs=*/
  |u| : Outport
  ∠u : Outport  Port=2
  wires:
  input signal/1 -> An Bn finder/1(signal)
  sin cos wave generator/2(sin) -> An Bn finder/4(sin)
  sin cos wave generator/1(cos) -> An Bn finder/3(cos)
  Variable Time Delay10/1 -> sin cos wave generator/2(clock)
  "time period "/1 -> Add/3
  Data Store Read/1 -> Variable Time Delay10/2, Add/2
  Multiply/1 -> Product/1, An Bn finder/2(pulse)
  Product/1 -> sin cos wave generator/1(freq)
  Clock/1 -> Add/1
  Add/1 -> Sign/1
  Constant/1 -> "time period "/1
  Step/1 -> Add1/1
  Sign/1 -> Add1/2
  Pulse Generator/1 -> Add1/3
  Clock2/1 -> Variable Time Delay10/1
  Add1/1 -> Multiply/1
  Product1/1 -> Product/2
  An Bn finder/2(Bn) -> phase/2(Bn), magnitude/2(Bn)
  An Bn finder/1(An) -> phase/1(An), magnitude/1(An)
  magnitude/1(Out1) -> |u|/1
  phase/1(Out1) -> ∠u/1
  nth harmonics/1 -> Product1/2
  harmonic freq/1 -> An Bn finder/5("freq "), "time period "/2, Product1/1

== system HARMALYZE_model_simulink/Subsystem2/Subsystem3 ==
  input signal : Inport
  harmonic freq : Inport  Port=2
  nth harmonics : Inport  Port=3
  Add : Sum  Inputs=-++
  Add1 : Sum  Inputs=++-
  An Bn finder : Subsystem
  Clock : Clock
  Clock2 : Clock
  Constant : Constant
  Data Store Read : DataStoreRead  DataStoreName=delay
  Multiply : Gain  Gain=0.5
  Product : Product
  Product1 : Product
  Pulse Generator : DiscretePulseGenerator  PulseType=Time based  Period=4  PulseWidth=50
  Sign : Signum
  Step : Step  Time=2  SampleTime=0
  Variable Time Delay10 : VariableTransportDelay  MaximumDelay=10
  magnitude : Subsystem
  phase : Subsystem
  sin cos wave generator : Subsystem
  "time period " : Product  Inputs=*/
  |u| : Outport
  ∠u : Outport  Port=2
  wires:
  harmonic freq/1 -> Product1/1, "time period "/2, An Bn finder/5("freq ")
  nth harmonics/1 -> Product1/2
  phase/1(Out1) -> ∠u/1
  magnitude/1(Out1) -> |u|/1
  An Bn finder/1(An) -> magnitude/1(An), phase/1(An)
  An Bn finder/2(Bn) -> magnitude/2(Bn), phase/2(Bn)
  Product1/1 -> Product/2
  Add1/1 -> Multiply/1
  Clock2/1 -> Variable Time Delay10/1
  Pulse Generator/1 -> Add1/3
  Sign/1 -> Add1/2
  Step/1 -> Add1/1
  Constant/1 -> "time period "/1
  Add/1 -> Sign/1
  Clock/1 -> Add/1
  Product/1 -> sin cos wave generator/1(freq)
  Multiply/1 -> An Bn finder/2(pulse), Product/1
  Data Store Read/1 -> Add/2, Variable Time Delay10/2
  "time period "/1 -> Add/3
  Variable Time Delay10/1 -> sin cos wave generator/2(clock)
  sin cos wave generator/1(cos) -> An Bn finder/3(cos)
  sin cos wave generator/2(sin) -> An Bn finder/4(sin)
  input signal/1 -> An Bn finder/1(signal)

== system HARMALYZE_model_simulink/Subsystem2/Subsystem4 ==
  input signal : Inport
  harmonic freq : Inport  Port=2
  nth harmonics : Inport  Port=3
  Add : Sum  Inputs=-++
  Add1 : Sum  Inputs=++-
  An Bn finder : Subsystem
  Clock : Clock
  Clock2 : Clock
  Constant : Constant
  Data Store Read : DataStoreRead  DataStoreName=delay
  Multiply : Gain  Gain=0.5
  Product : Product
  Product1 : Product
  Pulse Generator : DiscretePulseGenerator  PulseType=Time based  Period=4  PulseWidth=50
  Sign : Signum
  Step : Step  Time=2  SampleTime=0
  Variable Time Delay10 : VariableTransportDelay  MaximumDelay=10
  magnitude : Subsystem
  phase : Subsystem
  sin cos wave generator : Subsystem
  "time period " : Product  Inputs=*/
  |u| : Outport
  ∠u : Outport  Port=2
  wires:
  input signal/1 -> An Bn finder/1(signal)
  sin cos wave generator/2(sin) -> An Bn finder/4(sin)
  sin cos wave generator/1(cos) -> An Bn finder/3(cos)
  Variable Time Delay10/1 -> sin cos wave generator/2(clock)
  "time period "/1 -> Add/3
  Data Store Read/1 -> Variable Time Delay10/2, Add/2
  Multiply/1 -> Product/1, An Bn finder/2(pulse)
  Product/1 -> sin cos wave generator/1(freq)
  Clock/1 -> Add/1
  Add/1 -> Sign/1
  Constant/1 -> "time period "/1
  Step/1 -> Add1/1
  Sign/1 -> Add1/2
  Pulse Generator/1 -> Add1/3
  Clock2/1 -> Variable Time Delay10/1
  Add1/1 -> Multiply/1
  Product1/1 -> Product/2
  An Bn finder/2(Bn) -> phase/2(Bn), magnitude/2(Bn)
  An Bn finder/1(An) -> phase/1(An), magnitude/1(An)
  magnitude/1(Out1) -> |u|/1
  phase/1(Out1) -> ∠u/1
  nth harmonics/1 -> Product1/2
  harmonic freq/1 -> An Bn finder/5("freq "), "time period "/2, Product1/1

== system HARMALYZE_model_simulink/Subsystem2/Subsystem5 ==
  input signal : Inport
  harmonic freq : Inport  Port=2
  nth harmonics : Inport  Port=3
  Add : Sum  Inputs=-++
  Add1 : Sum  Inputs=++-
  An Bn finder : Subsystem
  Clock : Clock
  Clock2 : Clock
  Constant : Constant
  Data Store Read : DataStoreRead  DataStoreName=delay
  Multiply : Gain  Gain=0.5
  Product : Product
  Product1 : Product
  Pulse Generator : DiscretePulseGenerator  PulseType=Time based  Period=4  PulseWidth=50
  Sign : Signum
  Step : Step  Time=2  SampleTime=0
  Variable Time Delay10 : VariableTransportDelay  MaximumDelay=10
  magnitude : Subsystem
  phase : Subsystem
  sin cos wave generator : Subsystem
  "time period " : Product  Inputs=*/
  |u| : Outport
  ∠u : Outport  Port=2
  wires:
  input signal/1 -> An Bn finder/1(signal)
  sin cos wave generator/2(sin) -> An Bn finder/4(sin)
  sin cos wave generator/1(cos) -> An Bn finder/3(cos)
  Variable Time Delay10/1 -> sin cos wave generator/2(clock)
  "time period "/1 -> Add/3
  Data Store Read/1 -> Variable Time Delay10/2, Add/2
  Multiply/1 -> Product/1, An Bn finder/2(pulse)
  Product/1 -> sin cos wave generator/1(freq)
  Clock/1 -> Add/1
  Add/1 -> Sign/1
  Constant/1 -> "time period "/1
  Step/1 -> Add1/1
  Sign/1 -> Add1/2
  Pulse Generator/1 -> Add1/3
  Clock2/1 -> Variable Time Delay10/1
  Add1/1 -> Multiply/1
  Product1/1 -> Product/2
  An Bn finder/2(Bn) -> phase/2(Bn), magnitude/2(Bn)
  An Bn finder/1(An) -> phase/1(An), magnitude/1(An)
  magnitude/1(Out1) -> |u|/1
  phase/1(Out1) -> ∠u/1
  nth harmonics/1 -> Product1/2
  harmonic freq/1 -> An Bn finder/5("freq "), "time period "/2, Product1/1

== system HARMALYZE_model_simulink/Subsystem2/Subsystem6 ==
  input signal : Inport
  harmonic freq : Inport  Port=2
  nth harmonics : Inport  Port=3
  Add : Sum  Inputs=-++
  Add1 : Sum  Inputs=++-
  An Bn finder : Subsystem
  Clock : Clock
  Clock2 : Clock
  Constant : Constant
  Data Store Read : DataStoreRead  DataStoreName=delay
  Multiply : Gain  Gain=0.5
  Product : Product
  Product1 : Product
  Pulse Generator : DiscretePulseGenerator  PulseType=Time based  Period=4  PulseWidth=50
  Sign : Signum
  Step : Step  Time=2  SampleTime=0
  Variable Time Delay10 : VariableTransportDelay  MaximumDelay=10
  magnitude : Subsystem
  phase : Subsystem
  sin cos wave generator : Subsystem
  "time period " : Product  Inputs=*/
  |u| : Outport
  ∠u : Outport  Port=2
  wires:
  input signal/1 -> An Bn finder/1(signal)
  sin cos wave generator/2(sin) -> An Bn finder/4(sin)
  sin cos wave generator/1(cos) -> An Bn finder/3(cos)
  Variable Time Delay10/1 -> sin cos wave generator/2(clock)
  "time period "/1 -> Add/3
  Data Store Read/1 -> Variable Time Delay10/2, Add/2
  Multiply/1 -> Product/1, An Bn finder/2(pulse)
  Product/1 -> sin cos wave generator/1(freq)
  Clock/1 -> Add/1
  Add/1 -> Sign/1
  Constant/1 -> "time period "/1
  Step/1 -> Add1/1
  Sign/1 -> Add1/2
  Pulse Generator/1 -> Add1/3
  Clock2/1 -> Variable Time Delay10/1
  Add1/1 -> Multiply/1
  Product1/1 -> Product/2
  An Bn finder/2(Bn) -> phase/2(Bn), magnitude/2(Bn)
  An Bn finder/1(An) -> phase/1(An), magnitude/1(An)
  magnitude/1(Out1) -> |u|/1
  phase/1(Out1) -> ∠u/1
  nth harmonics/1 -> Product1/2
  harmonic freq/1 -> An Bn finder/5("freq "), "time period "/2, Product1/1

== system HARMALYZE_model_simulink/Subsystem2/Subsystem7 ==
  input signal : Inport
  harmonic freq : Inport  Port=2
  nth harmonics : Inport  Port=3
  Add : Sum  Inputs=-++
  Add1 : Sum  Inputs=++-
  An Bn finder : Subsystem
  Clock : Clock
  Clock2 : Clock
  Constant : Constant
  Data Store Read : DataStoreRead  DataStoreName=delay
  Multiply : Gain  Gain=0.5
  Product : Product
  Product1 : Product
  Pulse Generator : DiscretePulseGenerator  PulseType=Time based  Period=4  PulseWidth=50
  Sign : Signum
  Step : Step  Time=2  SampleTime=0
  Variable Time Delay10 : VariableTransportDelay  MaximumDelay=10
  magnitude : Subsystem
  phase : Subsystem
  sin cos wave generator : Subsystem
  "time period " : Product  Inputs=*/
  |u| : Outport
  ∠u : Outport  Port=2
  wires:
  input signal/1 -> An Bn finder/1(signal)
  sin cos wave generator/2(sin) -> An Bn finder/4(sin)
  sin cos wave generator/1(cos) -> An Bn finder/3(cos)
  Variable Time Delay10/1 -> sin cos wave generator/2(clock)
  "time period "/1 -> Add/3
  Data Store Read/1 -> Variable Time Delay10/2, Add/2
  Multiply/1 -> Product/1, An Bn finder/2(pulse)
  Product/1 -> sin cos wave generator/1(freq)
  Clock/1 -> Add/1
  Add/1 -> Sign/1
  Constant/1 -> "time period "/1
  Step/1 -> Add1/1
  Sign/1 -> Add1/2
  Pulse Generator/1 -> Add1/3
  Clock2/1 -> Variable Time Delay10/1
  Add1/1 -> Multiply/1
  Product1/1 -> Product/2
  An Bn finder/2(Bn) -> phase/2(Bn), magnitude/2(Bn)
  An Bn finder/1(An) -> phase/1(An), magnitude/1(An)
  magnitude/1(Out1) -> |u|/1
  phase/1(Out1) -> ∠u/1
  nth harmonics/1 -> Product1/2
  harmonic freq/1 -> An Bn finder/5("freq "), "time period "/2, Product1/1

== system HARMALYZE_model_simulink/Subsystem2/Subsystem8 ==
  input signal : Inport
  harmonic freq : Inport  Port=2
  nth harmonics : Inport  Port=3
  Add : Sum  Inputs=-++
  Add1 : Sum  Inputs=++-
  An Bn finder : Subsystem
  Clock : Clock
  Clock2 : Clock
  Constant : Constant
  Data Store Read : DataStoreRead  DataStoreName=delay
  Multiply : Gain  Gain=0.5
  Product : Product
  Product1 : Product
  Pulse Generator : DiscretePulseGenerator  PulseType=Time based  Period=4  PulseWidth=50
  Sign : Signum
  Step : Step  Time=2  SampleTime=0
  Variable Time Delay10 : VariableTransportDelay  MaximumDelay=10
  magnitude : Subsystem
  phase : Subsystem
  sin cos wave generator : Subsystem
  "time period " : Product  Inputs=*/
  |u| : Outport
  ∠u : Outport  Port=2
  wires:
  harmonic freq/1 -> Product1/1, "time period "/2, An Bn finder/5("freq ")
  nth harmonics/1 -> Product1/2
  phase/1(Out1) -> ∠u/1
  magnitude/1(Out1) -> |u|/1
  An Bn finder/1(An) -> magnitude/1(An), phase/1(An)
  An Bn finder/2(Bn) -> magnitude/2(Bn), phase/2(Bn)
  Product1/1 -> Product/2
  Add1/1 -> Multiply/1
  Clock2/1 -> Variable Time Delay10/1
  Pulse Generator/1 -> Add1/3
  Sign/1 -> Add1/2
  Step/1 -> Add1/1
  Constant/1 -> "time period "/1
  Add/1 -> Sign/1
  Clock/1 -> Add/1
  Product/1 -> sin cos wave generator/1(freq)
  Multiply/1 -> An Bn finder/2(pulse), Product/1
  Data Store Read/1 -> Add/2, Variable Time Delay10/2
  "time period "/1 -> Add/3
  Variable Time Delay10/1 -> sin cos wave generator/2(clock)
  sin cos wave generator/1(cos) -> An Bn finder/3(cos)
  sin cos wave generator/2(sin) -> An Bn finder/4(sin)
  input signal/1 -> An Bn finder/1(signal)

== system HARMALYZE_model_simulink/Subsystem2/Subsystem9 ==
  input signal : Inport
  harmonic freq : Inport  Port=2
  nth harmonics : Inport  Port=3
  Add : Sum  Inputs=-++
  Add1 : Sum  Inputs=++-
  An Bn finder : Subsystem
  Clock : Clock
  Clock2 : Clock
  Constant : Constant
  Data Store Read : DataStoreRead  DataStoreName=delay
  Multiply : Gain  Gain=0.5
  Product : Product
  Product1 : Product
  Pulse Generator : DiscretePulseGenerator  PulseType=Time based  Period=4  PulseWidth=50
  Sign : Signum
  Step : Step  Time=2  SampleTime=0
  Variable Time Delay10 : VariableTransportDelay  MaximumDelay=10
  magnitude : Subsystem
  phase : Subsystem
  sin cos wave generator : Subsystem
  "time period " : Product  Inputs=*/
  |u| : Outport
  ∠u : Outport  Port=2
  wires:
  harmonic freq/1 -> Product1/1, "time period "/2, An Bn finder/5("freq ")
  nth harmonics/1 -> Product1/2
  phase/1(Out1) -> ∠u/1
  magnitude/1(Out1) -> |u|/1
  An Bn finder/1(An) -> magnitude/1(An), phase/1(An)
  An Bn finder/2(Bn) -> magnitude/2(Bn), phase/2(Bn)
  Product1/1 -> Product/2
  Add1/1 -> Multiply/1
  Clock2/1 -> Variable Time Delay10/1
  Pulse Generator/1 -> Add1/3
  Sign/1 -> Add1/2
  Step/1 -> Add1/1
  Constant/1 -> "time period "/1
  Add/1 -> Sign/1
  Clock/1 -> Add/1
  Product/1 -> sin cos wave generator/1(freq)
  Multiply/1 -> An Bn finder/2(pulse), Product/1
  Data Store Read/1 -> Add/2, Variable Time Delay10/2
  "time period "/1 -> Add/3
  Variable Time Delay10/1 -> sin cos wave generator/2(clock)
  sin cos wave generator/1(cos) -> An Bn finder/3(cos)
  sin cos wave generator/2(sin) -> An Bn finder/4(sin)
  input signal/1 -> An Bn finder/1(signal)

== system HARMALYZE_model_simulink/implementing PLL/If Action Subsystem ==
  In1 : Inport
  Action Port : ActionPort  ActionPortLabel=if(u1 == u2)
  Out1 : Outport
  wires:
  In1/1 -> Out1/1

== system HARMALYZE_model_simulink/Subsystem2/Subsystem/An Bn finder ==
  signal : Inport
  pulse : Inport  Port=2
  cos : Inport  Port=3
  sin : Inport  Port=4
  "freq " : Inport  Port=5
  Add2 : Sum  Inputs=+-
  Constant1 : Constant  Value=0.01
  Data Store Read1 : DataStoreRead  DataStoreName=simultion_time
  Product : Product  Inputs=3
  Product{1,3..5} (4 alike) : Product
  Product2 : Product  Inputs=3
  Pulse Generator1 : DiscretePulseGenerator  PulseType=Time based  Period=1  PulseWidth=0.01
  Transfer Fcn1 : TransferFcn  Numerator=[2]  Denominator=[1 0]
  Transfer Fcn2 : TransferFcn  Numerator=[2]  Denominator=[1 0]
  Variable Time Delay1 : VariableTransportDelay  MaximumDelay=10
  An : Outport
  Bn : Outport  Port=2
  wires:
  pulse/1 -> Product/1, Product2/2
  signal/1 -> Product2/1, Product/2
  Product/1 -> Transfer Fcn1/1
  Product2/1 -> Transfer Fcn2/1
  cos/1 -> Product/3
  sin/1 -> Product2/3
  Transfer Fcn2/1 -> Product3/2
  Transfer Fcn1/1 -> Product1/1
  "freq "/1 -> Product1/2, Product3/1
  Pulse Generator1/1 -> Variable Time Delay1/1
  Product1/1 -> Product5/1  "An"
  Constant1/1 -> Add2/2
  Data Store Read1/1 -> Add2/1
  Variable Time Delay1/1 -> Product5/2, Product4/1
  Add2/1 -> Variable Time Delay1/2
  Product3/1 -> Product4/2  "Bn"
  Product5/1 -> An/1
  Product4/1 -> Bn/1

== system HARMALYZE_model_simulink/Subsystem2/Subsystem/magnitude ==
  An : Inport
  Bn : Inport  Port=2
  Add3 : Sum
  Math Function : Math  Operator=square  SignedPower=off  SaturateOnIntegerOverflow=on
  Math Function1 : Math  Operator=square  SignedPower=off  SaturateOnIntegerOverflow=on
  Sqrt : Sqrt  SaturateOnIntegerOverflow=on
  Out1 : Outport
  wires:
  Math Function/1 -> Add3/1
  Add3/1 -> Sqrt/1
  Math Function1/1 -> Add3/2
  Sqrt/1 -> Out1/1
  Bn/1 -> Math Function1/1
  An/1 -> Math Function/1

== system HARMALYZE_model_simulink/Subsystem2/Subsystem/phase ==
  An : Inport
  Bn : Inport  Port=2
  Multiply1 : Gain  Gain=180/pi
  Sin : Trigonometry  Operator=atan2
  Out1 : Outport
  wires:
  Sin/1 -> Multiply1/1
  An/1 -> Sin/2
  Bn/1 -> Sin/1
  Multiply1/1 -> Out1/1

== system HARMALYZE_model_simulink/Subsystem2/Subsystem/sin cos wave generator ==
  freq : Inport
  clock : Inport  Port=2
  Cos1 : Trigonometry  Operator=cos
  Gain : Gain  Gain=2*pi
  Product1 : Product
  Sin1 : Trigonometry
  cos : Outport
  sin : Outport  Port=2
  wires:
  Cos1/1 -> cos/1
  freq/1 -> Product1/1
  clock/1 -> Product1/2
  Sin1/1 -> sin/1
  Product1/1 -> Gain/1
  Gain/1 -> Sin1/1, Cos1/1
